simulink model "hcu_main_ADASwEPS"  (Simulink 8.2)
settings: Solver=FixedStepDiscrete  StartTime=0.0  StopTime=inf  FixedStep=0.001  RelTol=1e-3
PostLoadFcn:
  | , if any(exist('dsrtsu_mdlpostloadfcn', 'file') == [2, 3, 6]), try dsrtsu_mdlpostloadfcn('Execute', bdroot); catch fprintf('Error in PostLoadFcn (dsrtsu_mdlpostloadfcn) for model "%s":\n %s\n', bdroot, lasterr); end, end,
values from neighbouring files (symbols this model uses):
  C_TASK_1MS_S = (	C_TICK_TIME_S       )    [hcu_local_hdr.m]    (also in temp_ovrd_values.m = double(	0.001                  ))
  C_TICK_TIME_S = single(	0.005	    	)    [hcu_local_hdr.m]
  ENUM_EPSLFCSTATUS_ACTIVE = uint8(  2  )    [hcu_local_hdr.m]
  ENUM_EPSLFCSTATUS_TRANSITION = uint8(  3  )    [hcu_local_hdr.m]
  ENUM_EPSLKASTATUS_ACTIVE = uint8(  2  )    [hcu_local_hdr.m]
  ENUM_EPSMODEREQ_ANGLE = uint8(  1  )    [hcu_local_hdr.m]
  ENUM_EPSMODEREQ_INTERNAL = uint8(  0  )    [hcu_local_hdr.m]
  ENUM_EPSMODEREQ_TORQUE = uint8(  2  )    [hcu_local_hdr.m]
  ENUM_GEARPOSN_1ST = uint8(  1  )    [hcu_local_hdr.m]
  ENUM_GEARPOSN_2ND = uint8(  2  )    [hcu_local_hdr.m]
  ENUM_GEARPOSN_3RD = uint8(  3  )    [hcu_local_hdr.m]
  ENUM_GEARPOSN_4TH = uint8(  4  )    [hcu_local_hdr.m]
  ENUM_GEARPOSN_5TH = uint8(  5  )    [hcu_local_hdr.m]
  ENUM_GEARPOSN_6TH = uint8(  6  )    [hcu_local_hdr.m]
  ENUM_GEARPOSN_R = uint8(  7  )    [hcu_local_hdr.m]
  FALSE = boolean( 0 )    [hcu_local_hdr.m]
  TRUE = boolean( 1 )    [hcu_local_hdr.m]
undefined symbols (not defined in the file or in its folder): AISP_EPSCurrent_pct, AISP_TqASensorDelta_pct, AISP_TqBSensorDelta_pct, dHAL_IN, hal, INVALID_ABS1_TIMEOUT, INVALID_ABS2_TIMEOUT, INVALID_ABS3_TIMEOUT, INVALID_ABS4_TIMEOUT, INVALID_AC1_TIMEOUT, INVALID_ADASTORQ_REQ, INVALID_BCM1_TIMEOUT, INVALID_BCM2_TIMEOUT, INVALID_BOOSTER_VAC, INVALID_CSW1_TIMEOUT, INVALID_CUR_VEHDECE, INVALID_CURBRAKEDECE_REQ, INVALID_CURSTEERANG_REQ, INVALID_CURSTEERTQ_REQ, INVALID_ECM1_TIMEOUT, INVALID_ECM2_TIMEOUT, INVALID_ECM3_TIMEOUT, INVALID_ECM9_TIMEOUT, INVALID_ENG_TORQUE_FRICTIONAL, INVALID_ENG_TORQUE_INDICATED, INVALID_ENG_TORQUE_INDICATEDCOR, INVALID_ENG_TQ_MAX, INVALID_ENG_TQ_MIN, INVALID_EPAS2_TIMEOUT, INVALID_EPAS3_TIMEOUT, INVALID_EPB1_TIMEOUT, INVALID_EPS_BATTVOLT, INVALID_ESC_BATTVOLT, INVALID_GRADE, INVALID_HCU3_TIMEOUT, INVALID_HCU4_TIMEOUT, INVALID_HMI1_TIMEOUT, INVALID_HMI2_TIMEOUT, INVALID_LAT_ACC, INVALID_LONG_ACC, INVALID_MC_PRESSURE, INVALID_METER1_TIMEOUT, INVALID_METER3_TIMEOUT, INVALID_METER_VEHSPD, INVALID_ODO_METER, INVALID_OUTSIDE_TEMP, INVALID_PARKBRAKEBIND_STAT, INVALID_PEDALTQ_REQ, INVALID_SAS1_TIMEOUT, INVALID_SAS_ANGLE, INVALID_SHIFTER_POSN, INVALID_TCM1_TIMEOUT, INVALID_TCM2_TIMEOUT, INVALID_VCU1_TIMEOUT, INVALID_VCU2_TIMEOUT, INVALID_VEH_CRASH, INVALID_VEH_SPD, INVALID_WHEEL_SPD, INVALID_YAW_RATE, KHAL_MssgIdObj1_num ... (+8)
libraries: simulink x147, hcu_lib x38, rti1401lib_dio_type3 x4, rtimmsu_dsrtlib x3, app x1, rtiethernetudplib x1, rti1401lib_adc_type4 x1, rti1401lib_dac_type3 x1, inp x1, lidr x1, outp x1
(part 10 of 15)

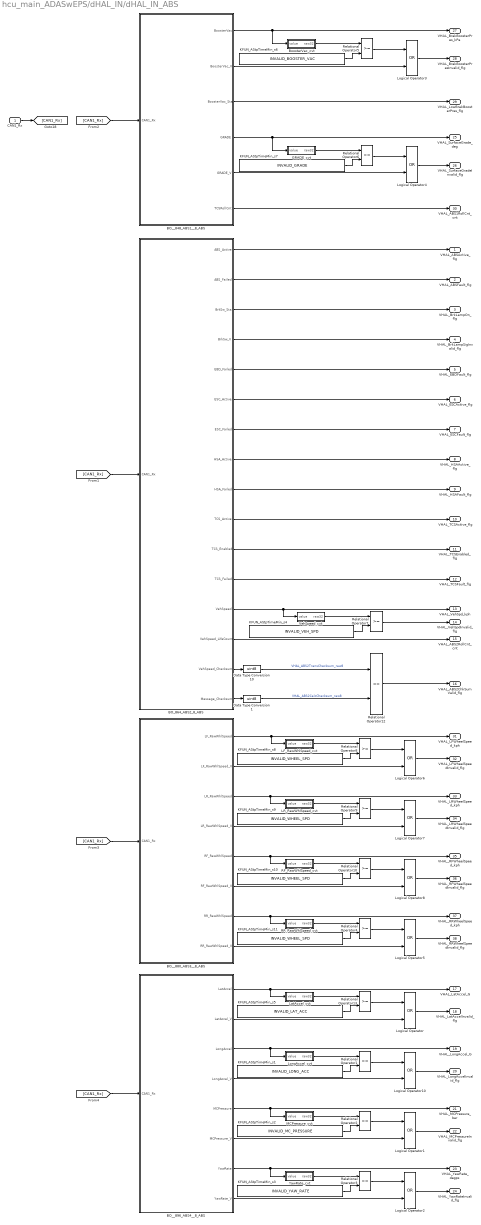
== system hcu_main_ADASwEPS/dHAL_IN/dHAL_IN_ABS ==
  CAN1_Rx : Inport
  BO_864_ABS2_8_ABS : Subsystem
  BO__848_ABS1__8_ABS : Subsystem
  BO__880_ABS3__8_ABS : Subsystem
  BO__896_ABS4__8_ABS : Subsystem
  BoosterVac_cvt : Subsystem  mask(ConvertOut){gain=0.3937, offset=0}
      mask help:
      | Conversion Formula
      |
      | The conversion formula is
      |
      | raw_value = (physical_value - Offset) / Factor
      |
      | where physical_value is the value of the signal after it is saturated using the specified Min and Max values. raw_value is the packed signal value.
  Data Type Conversion1 : DataTypeConversion  OutDataTypeStr=uint8
  Data Type Conversion10 : DataTypeConversion  OutDataTypeStr=uint8
  GRADE_cvt : Subsystem  mask(ConvertOut){gain=0.354331, offset=-45}
      mask help:
      | Conversion Formula
      |
      | The conversion formula is
      |
      | raw_value = (physical_value - Offset) / Factor
      |
      | where physical_value is the value of the signal after it is saturated using the specified Min and Max values. raw_value is the packed signal value.
  KFUN_AStpTimeMin_s1 : Constant  Value=INVALID_LONG_ACC
  KFUN_AStpTimeMin_s{8..11} (4 alike) : Constant  Value=INVALID_WHEEL_SPD
  KFUN_AStpTimeMin_s2 : Constant  Value=INVALID_MC_PRESSURE
  KFUN_AStpTimeMin_s3 : Constant  Value=INVALID_YAW_RATE
  KFUN_AStpTimeMin_s4 : Constant  Value=INVALID_VEH_SPD
  KFUN_AStpTimeMin_s5 : Constant  Value=INVALID_LAT_ACC
  KFUN_AStpTimeMin_s6 : Constant  Value=INVALID_BOOSTER_VAC
  KFUN_AStpTimeMin_s7 : Constant  Value=INVALID_GRADE
  LF_RawWhlSpeed_cvt : Subsystem  mask(ConvertOut){gain=0.015625, offset=0}
      mask help:
      | Conversion Formula
      |
      | The conversion formula is
      |
      | raw_value = (physical_value - Offset) / Factor
      |
      | where physical_value is the value of the signal after it is saturated using the specified Min and Max values. raw_value is the packed signal value.
  LR_RawWhlSpeed_cvt : Subsystem  mask(ConvertOut){gain=0.015625, offset=0}
      mask help:
      | Conversion Formula
      |
      | The conversion formula is
      |
      | raw_value = (physical_value - Offset) / Factor
      |
      | where physical_value is the value of the signal after it is saturated using the specified Min and Max values. raw_value is the packed signal value.
  LatAccel_cvt : Subsystem  mask(ConvertOut){gain=0.01, offset=-1.27}
      mask help:
      | Conversion Formula
      |
      | The conversion formula is
      |
      | raw_value = (physical_value - Offset) / Factor
      |
      | where physical_value is the value of the signal after it is saturated using the specified Min and Max values. raw_value is the packed signal value.
  Logical Operator{,1..8,10} (10 alike) : Logic  Operator=OR  AllPortsSameDT=off  OutDataTypeStr=boolean
  LongAccel_cvt : Subsystem  mask(ConvertOut){gain=0.01, offset=-1.27}
      mask help:
      | Conversion Formula
      |
      | The conversion formula is
      |
      | raw_value = (physical_value - Offset) / Factor
      |
      | where physical_value is the value of the signal after it is saturated using the specified Min and Max values. raw_value is the packed signal value.
  MCPressure_cvt : Subsystem  mask(ConvertOut){gain=0.1, offset=-11.6}
      mask help:
      | Conversion Formula
      |
      | The conversion formula is
      |
      | raw_value = (physical_value - Offset) / Factor
      |
      | where physical_value is the value of the signal after it is saturated using the specified Min and Max values. raw_value is the packed signal value.
  RF_RawWhlSpeed_cvt : Subsystem  mask(ConvertOut){gain=0.015625, offset=0}
      mask help:
      | Conversion Formula
      |
      | The conversion formula is
      |
      | raw_value = (physical_value - Offset) / Factor
      |
      | where physical_value is the value of the signal after it is saturated using the specified Min and Max values. raw_value is the packed signal value.
  RR_RawWhlSpeed_cvt : Subsystem  mask(ConvertOut){gain=0.015625, offset=0}
      mask help:
      | Conversion Formula
      |
      | The conversion formula is
      |
      | raw_value = (physical_value - Offset) / Factor
      |
      | where physical_value is the value of the signal after it is saturated using the specified Min and Max values. raw_value is the packed signal value.
  Relational Operator{1..10,13} (11 alike) : RelationalOperator  OutDataTypeStr=boolean
  Relational Operator12 : RelationalOperator  Operator===  OutDataTypeStr=boolean
  VehSpeed_cvt : Subsystem  mask(ConvertOut){gain=0.125, offset=0}
      mask help:
      | Conversion Formula
      |
      | The conversion formula is
      |
      | raw_value = (physical_value - Offset) / Factor
      |
      | where physical_value is the value of the signal after it is saturated using the specified Min and Max values. raw_value is the packed signal value.
  YawRate_cvt : Subsystem  mask(ConvertOut){gain=0.1, offset=-100}
      mask help:
      | Conversion Formula
      |
      | The conversion formula is
      |
      | raw_value = (physical_value - Offset) / Factor
      |
      | where physical_value is the value of the signal after it is saturated using the specified Min and Max values. raw_value is the packed signal value.
  VHAL_ABSActive_flg : Outport
  VHAL_ABSFault_flg : Outport  Port=2
  VHAL_BrkLampOn_flg : Outport  Port=3
  VHAL_BrkLampSigInvalid_flg : Outport  Port=4
  VHAL_EBDFault_flg : Outport  Port=5
  VHAL_ESCActive_flg : Outport  Port=6
  VHAL_ESCFault_flg : Outport  Port=7
  VHAL_HSAActive_flg : Outport  Port=8
  VHAL_HSAFault_flg : Outport  Port=9
  VHAL_TCSActive_flg : Outport  Port=10
  VHAL_TCSEnabled_flg : Outport  Port=11
  VHAL_TCSFault_flg : Outport  Port=12
  VHAL_VehSpd_kph : Outport  Port=13
  VHAL_VehSpdInvalid_flg : Outport  Port=14
  VHAL_ABS2RollCnt_cnt : Outport  Port=15
  VHAL_ABS2ChkSumValid_flg : Outport  Port=16
  VHAL_LatAccel_G : Outport  Port=17
  VHAL_LatAccelInvalid_flg : Outport  Port=18
  VHAL_LongAccel_G : Outport  Port=19
  VHAL_LongAccelInvalid_flg : Outport  Port=20
  VHAL_MCPressure_bar : Outport  Port=21
  VHAL_MCPressureInvalid_flg : Outport  Port=22
  VHAL_YawRate_degps : Outport  Port=23
  VHAL_YawRateInvalid_flg : Outport  Port=24
  VHAL_SurfaceGrade_deg : Outport  Port=25
  VHAL_SurfaceGradeInvalid_flg : Outport  Port=26
  VHAL_BrakBoosterPres_kPa : Outport  Port=27
  VHAL_BrakBoosterPresInvalid_flg : Outport  Port=28
  VHAL_LowBrakBoosterPres_flg : Outport  Port=29
  VHAL_ABS1RollCnt_cnt : Outport  Port=30
  VHAL_LFWheelSpeed_kph : Outport  Port=31
  VHAL_LFWheelSpeedInvalid_flg : Outport  Port=32
  VHAL_LRWheelSpeed_kph : Outport  Port=33
  VHAL_LRWheelSpeedInvalid_flg : Outport  Port=34
  VHAL_RFWheelSpeed_kph : Outport  Port=35
  VHAL_RFWheelSpeedInvalid_flg : Outport  Port=36
  VHAL_RRWheelSpeed_kph : Outport  Port=37
  VHAL_RRWheelSpeedInvalid_flg : Outport  Port=38
  wires:
  BO_864_ABS2_8_ABS/1(ABS_Active) -> VHAL_ABSActive_flg/1
  BO_864_ABS2_8_ABS/2(ABS_Failed) -> VHAL_ABSFault_flg/1
  BO_864_ABS2_8_ABS/3(BrkSw_Sta) -> VHAL_BrkLampOn_flg/1
  BO_864_ABS2_8_ABS/4(BrkSw_V) -> VHAL_BrkLampSigInvalid_flg/1
  BO_864_ABS2_8_ABS/5(EBD_Failed) -> VHAL_EBDFault_flg/1
  BO_864_ABS2_8_ABS/6(ESC_Active) -> VHAL_ESCActive_flg/1
  BO_864_ABS2_8_ABS/7(ESC_Failed) -> VHAL_ESCFault_flg/1
  BO_864_ABS2_8_ABS/10(TCS_Active) -> VHAL_TCSActive_flg/1
  BO_864_ABS2_8_ABS/11(TCS_Enabled) -> VHAL_TCSEnabled_flg/1
  BO_864_ABS2_8_ABS/12(TCS_Failed) -> VHAL_TCSFault_flg/1
  BO__848_ABS1__8_ABS/6(TCSRollCnt) -> VHAL_ABS1RollCnt_cnt/1
  BO__896_ABS4__8_ABS/2(LatAccel_V) -> Logical Operator/2
  BO__896_ABS4__8_ABS/6(MCPressure_V) -> Logical Operator1/2
  Logical Operator/1 -> VHAL_LatAccelInvalid_flg/1
  Logical Operator10/1 -> VHAL_LongAccelInvalid_flg/1
  Logical Operator1/1 -> VHAL_MCPressureInvalid_flg/1
  Logical Operator2/1 -> VHAL_YawRateInvalid_flg/1
  BO_864_ABS2_8_ABS/8(HSA_Active) -> VHAL_HSAActive_flg/1
  BO_864_ABS2_8_ABS/9(HSA_Failed) -> VHAL_HSAFault_flg/1
  BO__848_ABS1__8_ABS/3(BoosterVac_Sta) -> VHAL_LowBrakBoosterPres_flg/1
  BO__880_ABS3__8_ABS/8(RR_RawWhlSpeed_V) -> Logical Operator5/2
  Logical Operator5/1 -> VHAL_RRWheelSpeedInvalid_flg/1
  BO_864_ABS2_8_ABS/14(VehSpeed_LifeCount) -> VHAL_ABS2RollCnt_cnt/1
  BO_864_ABS2_8_ABS/15(VehSpeed_Checksum) -> Data Type Conversion10/1
  BO_864_ABS2_8_ABS/16(Message_Checksum) -> Data Type Conversion1/1
  Relational Operator12/1 -> VHAL_ABS2ChkSumValid_flg/1
  Data Type Conversion10/1 -> Relational Operator12/1  "VHAL_ABS2TransChecksum_raw8"
  Data Type Conversion1/1 -> Relational Operator12/2  "VHAL_ABS2CalcChecksum_raw8"
  CAN1_Rx/1 -> [CAN1_Rx]
  [CAN1_Rx] -> BO_864_ABS2_8_ABS/1(CAN1_Rx)
  [CAN1_Rx] -> BO__848_ABS1__8_ABS/1(CAN1_Rx)
  [CAN1_Rx] -> BO__880_ABS3__8_ABS/1(CAN1_Rx)
  [CAN1_Rx] -> BO__896_ABS4__8_ABS/1(CAN1_Rx)
  BO__896_ABS4__8_ABS/8(YawRate_V) -> Logical Operator2/2
  BO__896_ABS4__8_ABS/4(LongAccel_V) -> Logical Operator10/2
  BO__896_ABS4__8_ABS/1(LatAccel) -> LatAccel_cvt/1(value), VHAL_LatAccel_G/1
  KFUN_AStpTimeMin_s5/1 -> Relational Operator13/2
  LatAccel_cvt/1(raw32) -> Relational Operator13/1
  Relational Operator13/1 -> Logical Operator/1
  BO__896_ABS4__8_ABS/3(LongAccel) -> LongAccel_cvt/1(value), VHAL_LongAccel_G/1
  KFUN_AStpTimeMin_s1/1 -> Relational Operator1/2
  LongAccel_cvt/1(raw32) -> Relational Operator1/1
  Relational Operator1/1 -> Logical Operator10/1
  BO__896_ABS4__8_ABS/5(MCPressure) -> MCPressure_cvt/1(value), VHAL_MCPressure_bar/1
  KFUN_AStpTimeMin_s2/1 -> Relational Operator2/2
  MCPressure_cvt/1(raw32) -> Relational Operator2/1
  Relational Operator2/1 -> Logical Operator1/1
  BO__896_ABS4__8_ABS/7(YawRate) -> YawRate_cvt/1(value), VHAL_YawRate_degps/1
  KFUN_AStpTimeMin_s3/1 -> Relational Operator3/2
  YawRate_cvt/1(raw32) -> Relational Operator3/1
  Relational Operator3/1 -> Logical Operator2/1
  BO__848_ABS1__8_ABS/2(BoosterVac_V) -> Logical Operator3/2
  Logical Operator3/1 -> VHAL_BrakBoosterPresInvalid_flg/1
  BO__848_ABS1__8_ABS/1(BoosterVac) -> BoosterVac_cvt/1(value), VHAL_BrakBoosterPres_kPa/1
  KFUN_AStpTimeMin_s6/1 -> Relational Operator5/2
  BoosterVac_cvt/1(raw32) -> Relational Operator5/1
  Relational Operator5/1 -> Logical Operator3/1
  Logical Operator4/1 -> VHAL_SurfaceGradeInvalid_flg/1
  BO__848_ABS1__8_ABS/4(GRADE) -> GRADE_cvt/1(value), VHAL_SurfaceGrade_deg/1
  KFUN_AStpTimeMin_s7/1 -> Relational Operator6/2
  GRADE_cvt/1(raw32) -> Relational Operator6/1
  Relational Operator6/1 -> Logical Operator4/1
  BO__848_ABS1__8_ABS/5(GRADE_V) -> Logical Operator4/2
  BO_864_ABS2_8_ABS/13(VehSpeed) -> VehSpeed_cvt/1(value), VHAL_VehSpd_kph/1
  KFUN_AStpTimeMin_s4/1 -> Relational Operator7/2
  VehSpeed_cvt/1(raw32) -> Relational Operator7/1
  Relational Operator7/1 -> VHAL_VehSpdInvalid_flg/1
  BO__880_ABS3__8_ABS/7(RR_RawWhlSpeed) -> RR_RawWhlSpeed_cvt/1(value), VHAL_RRWheelSpeed_kph/1
  KFUN_AStpTimeMin_s11/1 -> Relational Operator4/2
  RR_RawWhlSpeed_cvt/1(raw32) -> Relational Operator4/1
  Relational Operator4/1 -> Logical Operator5/1
  BO__880_ABS3__8_ABS/5(RF_RawWhlSpeed) -> RF_RawWhlSpeed_cvt/1(value), VHAL_RFWheelSpeed_kph/1
  KFUN_AStpTimeMin_s10/1 -> Relational Operator10/2
  RF_RawWhlSpeed_cvt/1(raw32) -> Relational Operator10/1
  Relational Operator10/1 -> Logical Operator8/1
  BO__880_ABS3__8_ABS/6(RF_RawWhlSpeed_V) -> Logical Operator8/2
  Logical Operator8/1 -> VHAL_RFWheelSpeedInvalid_flg/1
  BO__880_ABS3__8_ABS/3(LR_RawWhlSpeed) -> LR_RawWhlSpeed_cvt/1(value), VHAL_LRWheelSpeed_kph/1
  KFUN_AStpTimeMin_s9/1 -> Relational Operator9/2
  LR_RawWhlSpeed_cvt/1(raw32) -> Relational Operator9/1
  Relational Operator9/1 -> Logical Operator7/1
  BO__880_ABS3__8_ABS/4(LR_RawWhlSpeed_V) -> Logical Operator7/2
  Logical Operator7/1 -> VHAL_LRWheelSpeedInvalid_flg/1
  BO__880_ABS3__8_ABS/1(LF_RawWhlSpeed) -> LF_RawWhlSpeed_cvt/1(value), VHAL_LFWheelSpeed_kph/1
  KFUN_AStpTimeMin_s8/1 -> Relational Operator8/2
  LF_RawWhlSpeed_cvt/1(raw32) -> Relational Operator8/1
  Relational Operator8/1 -> Logical Operator6/1
  Logical Operator6/1 -> VHAL_LFWheelSpeedInvalid_flg/1
  BO__880_ABS3__8_ABS/2(LF_RawWhlSpeed_V) -> Logical Operator6/2

== system hcu_main_ADASwEPS/dHAL_IN/dHAL_IN_AC ==
  CAN1_Rx : Inport
  BO__1120_AC1__8_AC : Subsystem
  KFUN_AStpTimeMin_s1 : Constant  Value=INVALID_OUTSIDE_TEMP
  Relational Operator4 : RelationalOperator  OutDataTypeStr=boolean
  Sta_Out_Temp_cvt : Subsystem  mask(ConvertOut){gain=1, offset=-40}
      mask help:
      | Conversion Formula
      |
      | The conversion formula is
      |
      | raw_value = (physical_value - Offset) / Factor
      |
      | where physical_value is the value of the signal after it is saturated using the specified Min and Max values. raw_value is the packed signal value.
  VHAL_OutsideTemp_degC : Outport
  VHAL_OutsideTempInvalid_flg : Outport  Port=2
  wires:
  CAN1_Rx/1 -> [CAN1_Rx]
  [CAN1_Rx] -> BO__1120_AC1__8_AC/1(CAN1_Rx)
  BO__1120_AC1__8_AC/1(Sta_Out_Temp) -> Sta_Out_Temp_cvt/1(value), VHAL_OutsideTemp_degC/1
  KFUN_AStpTimeMin_s1/1 -> Relational Operator4/2
  Sta_Out_Temp_cvt/1(raw32) -> Relational Operator4/1
  Relational Operator4/1 -> VHAL_OutsideTempInvalid_flg/1

== system hcu_main_ADASwEPS/dHAL_IN/dHAL_IN_BCM ==
  CAN1_Rx : Inport
  BO__1008_BCM2__8_BCM : Subsystem
  BO__1056_BCM1__8_BCM : Subsystem
  Compare To Constant : simulink/Logic and Bit Operations/Compare To Constant  relop===  const=5  OutDataTypeStr=boolean  ZeroCross=off
  Compare To Constant1 : simulink/Logic and Bit Operations/Compare To Constant  relop=~=  const=5  OutDataTypeStr=boolean  ZeroCross=off
  Compare To Constant2 : simulink/Logic and Bit Operations/Compare To Constant  relop=~=  const=0  OutDataTypeStr=boolean  ZeroCross=off
  KFUN_AStpTimeMin_s3 : Constant  Value=INVALID_VEH_CRASH
  Logical Operator : Logic  Operator=OR  AllPortsSameDT=off  OutDataTypeStr=boolean
  Logical Operator1 : Logic  AllPortsSameDT=off  OutDataTypeStr=boolean
  Relational Operator3 : RelationalOperator  Operator===  OutDataTypeStr=boolean
  VHAL_KeySwitchStatus_enum : Outport
  VHAL_TurnSignalSwL_flg : Outport  Port=2
  VHAL_TurnSignalSwR_flg : Outport  Port=3
  VHAL_DriverDoorOpen_flg : Outport  Port=4
  VHAL_PassengerDoorOpen_flg : Outport  Port=5
  VHAL_LRDoorOpen_flg : Outport  Port=6
  VHAL_RRDoorOpen_flg : Outport  Port=7
  VHAL_TailGateOpen_flg : Outport  Port=8
  VHAL_AnyDoorOpen_flg : Outport  Port=9
  VHAL_HazardLightSw_flg : Outport  Port=10
  VHAL_VehCrashed_flg : Outport  Port=11
  VHAL_VehCrashedInvalid_flg : Outport  Port=12
  wires:
  Logical Operator/1 -> VHAL_VehCrashedInvalid_flg/1
  Relational Operator3/1 -> Logical Operator/1
  KFUN_AStpTimeMin_s3/1 -> Relational Operator3/2
  Compare To Constant/1 -> VHAL_VehCrashed_flg/1
  BO__1008_BCM2__8_BCM/1(BCM_SRS_Crash_Info) -> Compare To Constant2/1, Compare To Constant1/1, Relational Operator3/1, Compare To Constant/1
  BO__1056_BCM1__8_BCM/3(BCM_Hazard_Sta) -> VHAL_HazardLightSw_flg/1
  BO__1056_BCM1__8_BCM/1(BCM_AllDrSw_Sta) -> VHAL_AnyDoorOpen_flg/1
  BO__1056_BCM1__8_BCM/10(BCM_TGateSw_Sta) -> VHAL_TailGateOpen_flg/1
  BO__1056_BCM1__8_BCM/8(BCM_RRDrSw_Sta) -> VHAL_RRDoorOpen_flg/1
  BO__1056_BCM1__8_BCM/5(BCM_LRDrSw_Sta) -> VHAL_LRDoorOpen_flg/1
  BO__1056_BCM1__8_BCM/7(BCM_PDrSw_Sta) -> VHAL_PassengerDoorOpen_flg/1
  BO__1056_BCM1__8_BCM/2(BCM_DDrSw_Sta) -> VHAL_DriverDoorOpen_flg/1
  BO__1056_BCM1__8_BCM/4(BCM_Key_Sta) -> VHAL_KeySwitchStatus_enum/1
  BO__1056_BCM1__8_BCM/9(BCM_RTurnLp_Sta) -> VHAL_TurnSignalSwR_flg/1
  BO__1056_BCM1__8_BCM/6(BCM_LTurnLp_Sta) -> VHAL_TurnSignalSwL_flg/1
  CAN1_Rx/1 -> [CAN1_Rx]
  [CAN1_Rx] -> BO__1056_BCM1__8_BCM/1(CAN1_Rx)
  [CAN1_Rx] -> BO__1008_BCM2__8_BCM/1(CAN1_Rx)
  Compare To Constant1/1 -> Logical Operator1/1
  Compare To Constant2/1 -> Logical Operator1/2
  Logical Operator1/1 -> Logical Operator/2

== system hcu_main_ADASwEPS/dHAL_IN/dHAL_IN_ECM ==
  CAN1_Rx : Inport
  BO_790_ECM1_8_ECM : Subsystem
  BO_809_ECM2_8_ECM : Subsystem
  BO_821_ECM3_8_ECM : Subsystem
  BO_875_ECM9_8_ECM : Subsystem
  CAN_TQFR_cvt : Subsystem  mask(ConvertOut){gain=1.96, offset=-100}
      mask help:
      | Conversion Formula
      |
      | The conversion formula is
      |
      | raw_value = (physical_value - Offset) / Factor
      |
      | where physical_value is the value of the signal after it is saturated using the specified Min and Max values. raw_value is the packed signal value.
  CAN_TQI_ACOR_cvt : Subsystem  mask(ConvertOut){gain=1.96, offset=-100}
      mask help:
      | Conversion Formula
      |
      | The conversion formula is
      |
      | raw_value = (physical_value - Offset) / Factor
      |
      | where physical_value is the value of the signal after it is saturated using the specified Min and Max values. raw_value is the packed signal value.
  CAN_TQI_cvt : Subsystem  mask(ConvertOut){gain=1.96, offset=-100}
      mask help:
      | Conversion Formula
      |
      | The conversion formula is
      |
      | raw_value = (physical_value - Offset) / Factor
      |
      | where physical_value is the value of the signal after it is saturated using the specified Min and Max values. raw_value is the packed signal value.
  EngTqMax_cvt : Subsystem  mask(ConvertOut){gain=0.0078, offset=-100}
      mask help:
      | Conversion Formula
      |
      | The conversion formula is
      |
      | raw_value = (physical_value - Offset) / Factor
      |
      | where physical_value is the value of the signal after it is saturated using the specified Min and Max values. raw_value is the packed signal value.
  EngTqMin_cvt : Subsystem  mask(ConvertOut){gain=0.0078, offset=-100}
      mask help:
      | Conversion Formula
      |
      | The conversion formula is
      |
      | raw_value = (physical_value - Offset) / Factor
      |
      | where physical_value is the value of the signal after it is saturated using the specified Min and Max values. raw_value is the packed signal value.
  KFUN_AStpTimeMin_s1 : Constant  Value=INVALID_ENG_TORQUE_INDICATED
  KFUN_AStpTimeMin_s2 : Constant  Value=INVALID_ENG_TORQUE_INDICATEDCOR
  KFUN_AStpTimeMin_s3 : Constant  Value=INVALID_ENG_TORQUE_FRICTIONAL
  KFUN_AStpTimeMin_s5 : Constant  Value=INVALID_ENG_TQ_MAX
  KFUN_AStpTimeMin_s6 : Constant  Value=INVALID_ENG_TQ_MIN
  Relational Operator{1..5} (5 alike) : RelationalOperator  OutDataTypeStr=boolean
  VHAL_AccelPedalPosn_pct : Outport
  VHAL_AccelPedalPosnInvalid_flg : Outport  Port=2
  VHAL_EffAccelPedalPosn_pct : Outport  Port=3
  VHAL_EffAccelPedalPosnInvalid_flg : Outport  Port=4
  VHAL_EngSpd_rpm : Outport  Port=5
  VHAL_EngSpdInvalid_flg : Outport  Port=6
  VHAL_EngTqIndicated_Nm : Outport  Port=7
  VHAL_EngTqIndicatedInvalid_flg : Outport  Port=8
  VHAL_EngTqIndicatedCOR_Nm : Outport  Port=9
  VHAL_EngTqIndicatedCORInvalid_flg : Outport  Port=10
  VHAL_EngTqUnCORFault_flg : Outport  Port=11
  VHAL_EngTqFriction_Nm : Outport  Port=12
  VHAL_EngTqFrictionInvalid_flg : Outport  Port=13
  VHAL_EngTqMax_Nm : Outport  Port=14
  VHAL_EngTqMaxInvalid_flg : Outport  Port=15
  VHAL_EngTqMin_Nm : Outport  Port=16
  VHAL_EngTqMinInvalid_flg : Outport  Port=17
  VHAL_EMSHybridOpState_enum : Outport  Port=18
  VHAL_EMSOpState_enum : Outport  Port=19
  VHAL_ECM9RollCnt_cnt : Outport  Port=20
  VHAL_EngHoodOpen_flg : Outport  Port=21
  VHAL_OBDWarnCycAchiv_flg : Outport  Port=22
  VHAL_OBDDriveCycAchiv_flg : Outport  Port=23
  wires:
  CAN1_Rx/1 -> [CAN1_Rx]
  [CAN1_Rx] -> BO_821_ECM3_8_ECM/1(CAN1_Rx)
  BO_821_ECM3_8_ECM/4(LV_CAN_ERRPVS) -> VHAL_EffAccelPedalPosnInvalid_flg/1
  BO_821_ECM3_8_ECM/3(LV_CAN_ERRPAS) -> VHAL_AccelPedalPosnInvalid_flg/1
  BO_821_ECM3_8_ECM/2(CAN_PV_EFC) -> VHAL_EffAccelPedalPosn_pct/1
  BO_821_ECM3_8_ECM/1(CAN_PV_AV) -> VHAL_AccelPedalPosn_pct/1
  [CAN1_Rx] -> BO_790_ECM1_8_ECM/1(CAN1_Rx)
  BO_790_ECM1_8_ECM/6(LV_CAN_SUB_TQI) -> VHAL_EngTqUnCORFault_flg/1
  Relational Operator2/1 -> VHAL_EngTqIndicatedCORInvalid_flg/1
  BO_790_ECM1_8_ECM/4(CAN_TQI_ACOR) -> VHAL_EngTqIndicatedCOR_Nm/1, CAN_TQI_ACOR_cvt/1(value)
  BO_790_ECM1_8_ECM/3(CAN_TQI) -> VHAL_EngTqIndicated_Nm/1, CAN_TQI_cvt/1(value)
  Relational Operator1/1 -> VHAL_EngTqIndicatedInvalid_flg/1
  BO_790_ECM1_8_ECM/1(CAN_N) -> VHAL_EngSpd_rpm/1
  BO_790_ECM1_8_ECM/5(LV_CAN_N_ERR) -> VHAL_EngSpdInvalid_flg/1
  BO_790_ECM1_8_ECM/2(CAN_TQFR) -> VHAL_EngTqFriction_Nm/1, CAN_TQFR_cvt/1(value)
  Relational Operator3/1 -> VHAL_EngTqFrictionInvalid_flg/1
  [CAN1_Rx] -> BO_875_ECM9_8_ECM/1(CAN1_Rx1)
  BO_875_ECM9_8_ECM/3(EMSOpState) -> VHAL_EMSOpState_enum/1
  BO_875_ECM9_8_ECM/2(EMSHybridOpState) -> VHAL_EMSHybridOpState_enum/1
  BO_875_ECM9_8_ECM/1(ECM9RollCnt) -> VHAL_ECM9RollCnt_cnt/1
  [CAN1_Rx] -> BO_809_ECM2_8_ECM/1(CAN1_Rx)
  BO_809_ECM2_8_ECM/2(CAN_OBD_STAT_WU) -> VHAL_OBDWarnCycAchiv_flg/1
  BO_809_ECM2_8_ECM/1(Eng_Hood_SW) -> VHAL_EngHoodOpen_flg/1
  KFUN_AStpTimeMin_s2/1 -> Relational Operator2/2
  KFUN_AStpTimeMin_s1/1 -> Relational Operator1/2
  KFUN_AStpTimeMin_s3/1 -> Relational Operator3/2
  CAN_TQFR_cvt/1(raw32) -> Relational Operator3/1
  CAN_TQI_cvt/1(raw32) -> Relational Operator1/1
  CAN_TQI_ACOR_cvt/1(raw32) -> Relational Operator2/1
  Relational Operator4/1 -> VHAL_EngTqMaxInvalid_flg/1
  BO_875_ECM9_8_ECM/4(EngTqMax) -> EngTqMax_cvt/1(value), VHAL_EngTqMax_Nm/1
  KFUN_AStpTimeMin_s5/1 -> Relational Operator4/2
  EngTqMax_cvt/1(raw32) -> Relational Operator4/1
  Relational Operator5/1 -> VHAL_EngTqMinInvalid_flg/1
  BO_875_ECM9_8_ECM/5(EngTqMin) -> EngTqMin_cvt/1(value), VHAL_EngTqMin_Nm/1
  KFUN_AStpTimeMin_s6/1 -> Relational Operator5/2
  EngTqMin_cvt/1(raw32) -> Relational Operator5/1
  BO_809_ECM2_8_ECM/3(CAN_OBD_STAT_DR) -> VHAL_OBDDriveCycAchiv_flg/1

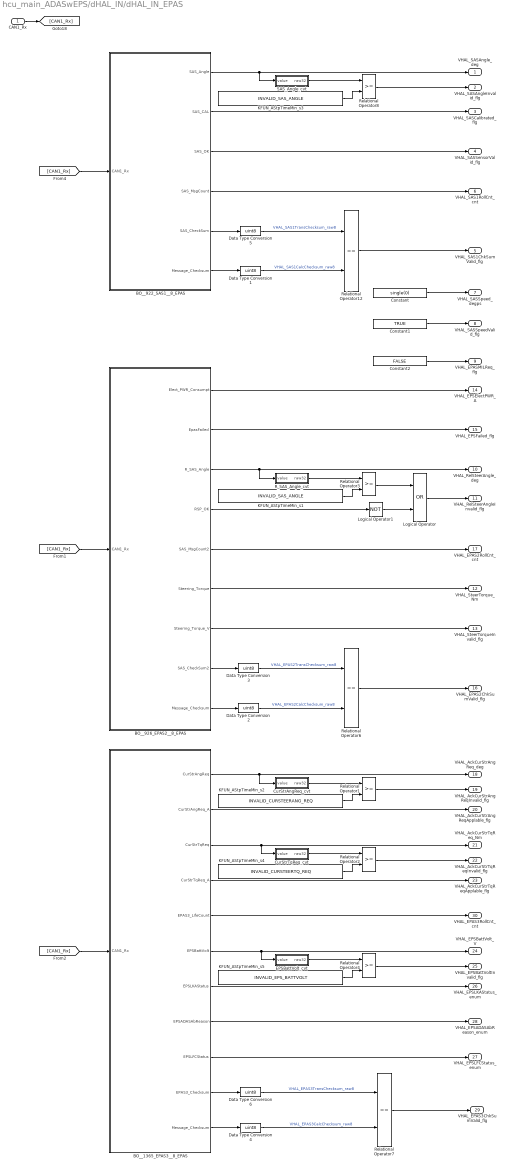
== system hcu_main_ADASwEPS/dHAL_IN/dHAL_IN_EPAS ==
  CAN1_Rx : Inport
  BO__1365_EPAS3__8_EPAS : Subsystem
  BO__922_SAS1__8_EPAS : Subsystem
  BO__926_EPAS2__8_EPAS : Subsystem
  Constant : Constant  Value=single(0)
  Constant1 : Constant  Value=TRUE
  Constant2 : Constant  Value=FALSE
  CurStrAngReq_cvt : Subsystem  mask(ConvertOut){gain=0.1, offset=-720}
      mask help:
      | Conversion Formula
      |
      | The conversion formula is
      |
      | raw_value = (physical_value - Offset) / Factor
      |
      | where physical_value is the value of the signal after it is saturated using the specified Min and Max values. raw_value is the packed signal value.
  CurStrTqReq_cvt : Subsystem  mask(ConvertOut){gain=0.1, offset=-10}
      mask help:
      | Conversion Formula
      |
      | The conversion formula is
      |
      | raw_value = (physical_value - Offset) / Factor
      |
      | where physical_value is the value of the signal after it is saturated using the specified Min and Max values. raw_value is the packed signal value.
  Data Type Conversion{1..6} (6 alike) : DataTypeConversion  OutDataTypeStr=uint8
  EPSBattVolt_cvt : Subsystem  mask(ConvertOut){gain=0.1, offset=0}
      mask help:
      | Conversion Formula
      |
      | The conversion formula is
      |
      | raw_value = (physical_value - Offset) / Factor
      |
      | where physical_value is the value of the signal after it is saturated using the specified Min and Max values. raw_value is the packed signal value.
  KFUN_AStpTimeMin_s1 : Constant  Value=INVALID_SAS_ANGLE
  KFUN_AStpTimeMin_s2 : Constant  Value=INVALID_CURSTEERANG_REQ
  KFUN_AStpTimeMin_s3 : Constant  Value=INVALID_SAS_ANGLE
  KFUN_AStpTimeMin_s4 : Constant  Value=INVALID_CURSTEERTQ_REQ
  KFUN_AStpTimeMin_s5 : Constant  Value=INVALID_EPS_BATTVOLT
  Logical Operator : Logic  Operator=OR  AllPortsSameDT=off  OutDataTypeStr=boolean
  Logical Operator1 : Logic  Operator=NOT  AllPortsSameDT=off  OutDataTypeStr=boolean
  R_SAS_Angle_cvt : Subsystem  mask(ConvertOut){gain=0.1, offset=-1400}
      mask help:
      | Conversion Formula
      |
      | The conversion formula is
      |
      | raw_value = (physical_value - Offset) / Factor
      |
      | where physical_value is the value of the signal after it is saturated using the specified Min and Max values. raw_value is the packed signal value.
  Relational Operator{1..4,8} (5 alike) : RelationalOperator  OutDataTypeStr=boolean
  Relational Operator12 : RelationalOperator  Operator===  OutDataTypeStr=boolean
  Relational Operator6 : RelationalOperator  Operator===  OutDataTypeStr=boolean
  Relational Operator7 : RelationalOperator  Operator===  OutDataTypeStr=boolean
  SAS_Angle_cvt : Subsystem  mask(ConvertOut){gain=0.1, offset=-900}
      mask help:
      | Conversion Formula
      |
      | The conversion formula is
      |
      | raw_value = (physical_value - Offset) / Factor
      |
      | where physical_value is the value of the signal after it is saturated using the specified Min and Max values. raw_value is the packed signal value.
  VHAL_SASAngle_deg : Outport
  VHAL_SASAngleInvalid_flg : Outport  Port=2
  VHAL_SASCalibrated_flg : Outport  Port=3
  VHAL_SASSensorValid_flg : Outport  Port=4
  VHAL_SAS1ChkSumValid_flg : Outport  Port=5
  VHAL_SAS1RollCnt_cnt : Outport  Port=6
  VHAL_SASSpeed_degps : Outport  Port=7
  VHAL_SASSpeedValid_flg : Outport  Port=8
  VHAL_EPASMILReq_flg : Outport  Port=9
  VHAL_RelSteerAngle_deg : Outport  Port=10
  VHAL_RelSteerAngleInvalid_flg : Outport  Port=11
  VHAL_SteerTorque_Nm : Outport  Port=12
  VHAL_SteerTorqueInvalid_flg : Outport  Port=13
  VHAL_EPSElectPWR_A : Outport  Port=14
  VHAL_EPSFailed_flg : Outport  Port=15
  VHAL_EPAS2ChkSumValid_flg : Outport  Port=16
  VHAL_EPAS2RollCnt_cnt : Outport  Port=17
  VHAL_AckCurStrAngReq_deg : Outport  Port=18
  VHAL_AckCurStrAngReqInvalid_flg : Outport  Port=19
  VHAL_AckCurStrAngReqApplable_flg : Outport  Port=20
  VHAL_AckCurStrTqReq_Nm : Outport  Port=21
  VHAL_AckCurStrTqReqInvalid_flg : Outport  Port=22
  VHAL_AckCurStrTqReqApplable_flg : Outport  Port=23
  VHAL_EPSBattVolt_V : Outport  Port=24
  VHAL_EPSBattVoltInvalid_flg : Outport  Port=25
  VHAL_EPSLKAStatus_enum : Outport  Port=26
  VHAL_EPSLFCStatus_enum : Outport  Port=27
  VHAL_EPSADASAbReason_enum : Outport  Port=28
  VHAL_EPAS3ChkSumValid_flg : Outport  Port=29
  VHAL_EPAS3RollCnt_cnt : Outport  Port=30
  wires:
  Constant2/1 -> VHAL_EPASMILReq_flg/1
  Constant1/1 -> VHAL_SASSpeedValid_flg/1
  Constant/1 -> VHAL_SASSpeed_degps/1
  BO__922_SAS1__8_EPAS/2(SAS_CAL) -> VHAL_SASCalibrated_flg/1
  BO__922_SAS1__8_EPAS/4(SAS_MsgCount) -> VHAL_SAS1RollCnt_cnt/1
  BO__922_SAS1__8_EPAS/3(SAS_OK) -> VHAL_SASSensorValid_flg/1
  BO__1365_EPAS3__8_EPAS/5(EPAS3_LifeCount) -> VHAL_EPAS3RollCnt_cnt/1
  BO__926_EPAS2__8_EPAS/1(Elect_PWR_Consumpt) -> VHAL_EPSElectPWR_A/1
  BO__926_EPAS2__8_EPAS/2(EpasFailed) -> VHAL_EPSFailed_flg/1
  BO__926_EPAS2__8_EPAS/4(RSP_OK) -> Logical Operator1/1
  BO__926_EPAS2__8_EPAS/5(SAS_MsgCount2) -> VHAL_EPAS2RollCnt_cnt/1
  BO__926_EPAS2__8_EPAS/6(Steering_Torque) -> VHAL_SteerTorque_Nm/1
  BO__926_EPAS2__8_EPAS/7(Steering_Torque_V) -> VHAL_SteerTorqueInvalid_flg/1
  Logical Operator/1 -> VHAL_RelSteerAngleInvalid_flg/1
  Logical Operator1/1 -> Logical Operator/2
  BO__1365_EPAS3__8_EPAS/4(CurStrTqReq_A) -> VHAL_AckCurStrTqReqApplable_flg/1
  BO__922_SAS1__8_EPAS/5(SAS_CheckSum) -> Data Type Conversion5/1
  BO__922_SAS1__8_EPAS/6(Message_Checksum) -> Data Type Conversion1/1
  Data Type Conversion5/1 -> Relational Operator12/1  "VHAL_SAS1TransChecksum_raw8"
  Data Type Conversion1/1 -> Relational Operator12/2  "VHAL_SAS1CalcChecksum_raw8"
  Relational Operator12/1 -> VHAL_SAS1ChkSumValid_flg/1
  Data Type Conversion3/1 -> Relational Operator6/1  "VHAL_EPAS2TransChecksum_raw8"
  Data Type Conversion2/1 -> Relational Operator6/2  "VHAL_EPAS2CalcChecksum_raw8"
  Relational Operator6/1 -> VHAL_EPAS2ChkSumValid_flg/1
  BO__926_EPAS2__8_EPAS/8(SAS_CheckSum2) -> Data Type Conversion3/1
  BO__926_EPAS2__8_EPAS/9(Message_Checksum) -> Data Type Conversion2/1
  Data Type Conversion6/1 -> Relational Operator7/1  "VHAL_EPAS3TransChecksum_raw8"
  Data Type Conversion4/1 -> Relational Operator7/2  "VHAL_EPAS3CalcChecksum_raw8"
  Relational Operator7/1 -> VHAL_EPAS3ChkSumValid_flg/1
  BO__1365_EPAS3__8_EPAS/10(EPAS3_Checksum) -> Data Type Conversion6/1
  BO__1365_EPAS3__8_EPAS/11(Message_Checksum) -> Data Type Conversion4/1
  BO__1365_EPAS3__8_EPAS/2(CurStrAngReq_A) -> VHAL_AckCurStrAngReqApplable_flg/1
  CAN1_Rx/1 -> [CAN1_Rx]
  [CAN1_Rx] -> BO__922_SAS1__8_EPAS/1(CAN1_Rx)
  [CAN1_Rx] -> BO__926_EPAS2__8_EPAS/1(CAN1_Rx)
  [CAN1_Rx] -> BO__1365_EPAS3__8_EPAS/1(CAN1_Rx)
  BO__922_SAS1__8_EPAS/1(SAS_Angle) -> SAS_Angle_cvt/1(value), VHAL_SASAngle_deg/1
  KFUN_AStpTimeMin_s3/1 -> Relational Operator8/2
  SAS_Angle_cvt/1(raw32) -> Relational Operator8/1
  Relational Operator8/1 -> VHAL_SASAngleInvalid_flg/1
  BO__926_EPAS2__8_EPAS/3(R_SAS_Angle) -> R_SAS_Angle_cvt/1(value), VHAL_RelSteerAngle_deg/1
  KFUN_AStpTimeMin_s1/1 -> Relational Operator3/2
  R_SAS_Angle_cvt/1(raw32) -> Relational Operator3/1
  Relational Operator3/1 -> Logical Operator/1
  BO__1365_EPAS3__8_EPAS/1(CurStrAngReq) -> CurStrAngReq_cvt/1(value), VHAL_AckCurStrAngReq_deg/1
  KFUN_AStpTimeMin_s2/1 -> Relational Operator1/2
  CurStrAngReq_cvt/1(raw32) -> Relational Operator1/1
  Relational Operator1/1 -> VHAL_AckCurStrAngReqInvalid_flg/1
  BO__1365_EPAS3__8_EPAS/3(CurStrTqReq) -> CurStrTqReq_cvt/1(value), VHAL_AckCurStrTqReq_Nm/1
  KFUN_AStpTimeMin_s4/1 -> Relational Operator2/2
  CurStrTqReq_cvt/1(raw32) -> Relational Operator2/1
  Relational Operator2/1 -> VHAL_AckCurStrTqReqInvalid_flg/1
  BO__1365_EPAS3__8_EPAS/6(EPSBattVolt) -> EPSBattVolt_cvt/1(value), VHAL_EPSBattVolt_V/1
  KFUN_AStpTimeMin_s5/1 -> Relational Operator4/2
  EPSBattVolt_cvt/1(raw32) -> Relational Operator4/1
  Relational Operator4/1 -> VHAL_EPSBattVoltInvalid_flg/1
  BO__1365_EPAS3__8_EPAS/7(EPSLKAStatus) -> VHAL_EPSLKAStatus_enum/1
  BO__1365_EPAS3__8_EPAS/8(EPSADASAbReason) -> VHAL_EPSADASAbReason_enum/1
  BO__1365_EPAS3__8_EPAS/9(EPSLFCStatus) -> VHAL_EPSLFCStatus_enum/1

== system hcu_main_ADASwEPS/dHAL_IN/dHAL_IN_HWIO ==
  IgnitionVolt_V : Constant  Value=12
  VbatprotVolt_V : Constant  Value=12
  VHAL_IgnitionVolt_V : Outport
  VHAL_VbatprotVolt_V : Outport  Port=2
  wires:
  IgnitionVolt_V/1 -> VHAL_IgnitionVolt_V/1
  VbatprotVolt_V/1 -> VHAL_VbatprotVolt_V/1

== system hcu_main_ADASwEPS/dHAL_IN/dHAL_IN_LLSW ==
  ADCFault_enum : Constant  Value=0
  AppTime_ms : Constant
  BuzzerSwOnFltOpenCircuit_enum : Constant  Value=0
  BuzzerSwOnFltShortHigh_enum : Constant  Value=0
  BuzzerSwOnFltShortLow_enum : Constant  Value=0
  EEPROMFault_enum : Constant  Value=0
  LampBlueOnFltOpenCircuit_enum : Constant  Value=0
  LampBuleOnFltShortHigh_enum : Constant  Value=0
  LampBuleOnFltShortLow_enum : Constant  Value=0
  LampGreenOnFltOpenCircuit_enum : Constant  Value=0
  LampGreenOnFltShortHigh_enum : Constant  Value=0
  LampGreenOnFltShortLow_enum : Constant  Value=0
  LampRedOnFltOpenCircuit_enum : Constant  Value=0
  LampRedOnFltShortHigh_enum : Constant  Value=0
  LampRedOnFltShortLow_enum : Constant  Value=0
  LampYellowOnFltOpenCircuit_enum : Constant  Value=0
  LampYellowOnFltShortHigh_enum : Constant  Value=0
  LampYellowOnFltShortLow_enum : Constant  Value=0
  OBUBuzzerOnFltOpenCircuit_enum : Constant  Value=0
  OBUBuzzerOnFltShortHigh_enum : Constant  Value=0
  OBUBuzzerOnFltShortLow_enum : Constant  Value=0
  RAMFault_enum : Constant  Value=0
  ROMFault_enum : Constant  Value=0
  VREF1Fault_enum : Constant  Value=0
  VREF2Fault_enum : Constant  Value=0
  VHAL_AppTime_ms : Outport
  VHAL_ADCFault_enum : Outport  Port=2
  VHAL_EEPROMFault_enum : Outport  Port=3
  VHAL_RAMFault_enum : Outport  Port=4
  VHAL_ROMFault_enum : Outport  Port=5
  VHAL_VREF1Fault_enum : Outport  Port=6
  VHAL_VREF2Fault_enum : Outport  Port=7
  VHAL_BuzzerSwOnFltOpenCircuit_enum : Outport  Port=8
  VHAL_BuzzerSwOnFltShortHigh_enum : Outport  Port=9
  VHAL_BuzzerSwOnFltShortLow_enum : Outport  Port=10
  VHAL_OBUBuzzerOnFltOpenCircuit_enum : Outport  Port=11
  VHAL_OBUBuzzerOnFltShortHigh_enum : Outport  Port=12
  VHAL_OBUBuzzerOnFltShortLow_enum : Outport  Port=13
  VHAL_LampRedOnFltOpenCircuit_enum : Outport  Port=14
  VHAL_LampRedOnFltShortHigh_enum : Outport  Port=15
  VHAL_LampRedOnFltShortLow_enum : Outport  Port=16
  VHAL_LampBlueOnFltOpenCircuit_enum : Outport  Port=17
  VHAL_LampBuleOnFltShortHigh_enum : Outport  Port=18
  VHAL_LampBuleOnFltShortLow_enum : Outport  Port=19
  VHAL_LampGreenOnFltOpenCircuit_enum : Outport  Port=20
  VHAL_LampGreenOnFltShortHigh_enum : Outport  Port=21
  VHAL_LampGreenOnFltShortLow_enum : Outport  Port=22
  VHAL_LampYellowOnFltOpenCircuit_enum : Outport  Port=23
  VHAL_LampYellowOnFltShortHigh_enum : Outport  Port=24
  VHAL_LampYellowOnFltShortLow_enum : Outport  Port=25
  wires:
  VREF2Fault_enum/1 -> VHAL_VREF2Fault_enum/1
  VREF1Fault_enum/1 -> VHAL_VREF1Fault_enum/1
  ROMFault_enum/1 -> VHAL_ROMFault_enum/1
  RAMFault_enum/1 -> VHAL_RAMFault_enum/1
  EEPROMFault_enum/1 -> VHAL_EEPROMFault_enum/1
  AppTime_ms/1 -> VHAL_AppTime_ms/1
  ADCFault_enum/1 -> VHAL_ADCFault_enum/1
  BuzzerSwOnFltOpenCircuit_enum/1 -> VHAL_BuzzerSwOnFltOpenCircuit_enum/1
  BuzzerSwOnFltShortHigh_enum/1 -> VHAL_BuzzerSwOnFltShortHigh_enum/1
  BuzzerSwOnFltShortLow_enum/1 -> VHAL_BuzzerSwOnFltShortLow_enum/1
  OBUBuzzerOnFltOpenCircuit_enum/1 -> VHAL_OBUBuzzerOnFltOpenCircuit_enum/1
  OBUBuzzerOnFltShortHigh_enum/1 -> VHAL_OBUBuzzerOnFltShortHigh_enum/1
  OBUBuzzerOnFltShortLow_enum/1 -> VHAL_OBUBuzzerOnFltShortLow_enum/1
  LampRedOnFltOpenCircuit_enum/1 -> VHAL_LampRedOnFltOpenCircuit_enum/1
  LampRedOnFltShortHigh_enum/1 -> VHAL_LampRedOnFltShortHigh_enum/1
  LampRedOnFltShortLow_enum/1 -> VHAL_LampRedOnFltShortLow_enum/1
  LampBlueOnFltOpenCircuit_enum/1 -> VHAL_LampBlueOnFltOpenCircuit_enum/1
  LampBuleOnFltShortHigh_enum/1 -> VHAL_LampBuleOnFltShortHigh_enum/1
  LampBuleOnFltShortLow_enum/1 -> VHAL_LampBuleOnFltShortLow_enum/1
  LampGreenOnFltOpenCircuit_enum/1 -> VHAL_LampGreenOnFltOpenCircuit_enum/1
  LampGreenOnFltShortHigh_enum/1 -> VHAL_LampGreenOnFltShortHigh_enum/1
  LampGreenOnFltShortLow_enum/1 -> VHAL_LampGreenOnFltShortLow_enum/1
  LampYellowOnFltOpenCircuit_enum/1 -> VHAL_LampYellowOnFltOpenCircuit_enum/1
  LampYellowOnFltShortHigh_enum/1 -> VHAL_LampYellowOnFltShortHigh_enum/1
  LampYellowOnFltShortLow_enum/1 -> VHAL_LampYellowOnFltShortLow_enum/1

== system hcu_main_ADASwEPS/dHAL_IN/dHAL_IN_METER ==
  CAN1_Rx : Inport
  BO__1104_Meter1__8_Meter : Subsystem
  BO__1306_Meter3__8_Meter : Subsystem
  KFUN_AStpTimeMin_s1 : Constant  Value=INVALID_METER_VEHSPD
  KFUN_AStpTimeMin_s5 : Constant  Value=INVALID_ODO_METER
  Meter_Ind_VehSpeed_cvt : Subsystem  mask(ConvertOut){gain=0.125, offset=0}
      mask help:
      | Conversion Formula
      |
      | The conversion formula is
      |
      | raw_value = (physical_value - Offset) / Factor
      |
      | where physical_value is the value of the signal after it is saturated using the specified Min and Max values. raw_value is the packed signal value.
  ODOMETER_cvt : Subsystem  mask(ConvertOut){gain=1, offset=0}
      mask help:
      | Conversion Formula
      |
      | The conversion formula is
      |
      | raw_value = (physical_value - Offset) / Factor
      |
      | where physical_value is the value of the signal after it is saturated using the specified Min and Max values. raw_value is the packed signal value.
  Relational Operator1 : RelationalOperator  OutDataTypeStr=boolean
  Relational Operator4 : RelationalOperator  OutDataTypeStr=boolean
  VHAL_OdoMeter_km : Outport
  VHAL_OdoMeterInvalid_flg : Outport  Port=2
  VHAL_LowBrakeFluid_flg : Outport  Port=3
  VHAL_ParkBrakeOn_flg : Outport  Port=4
  VHAL_SeatBeltNOTFasten_flg : Outport  Port=5
  VHAL_MeterVehSpd_kph : Outport  Port=6
  VHAL_MeterVehSpdInvalid_flg : Outport  Port=7
  wires:
  BO__1104_Meter1__8_Meter/4(SeatBelt) -> VHAL_SeatBeltNOTFasten_flg/1
  BO__1104_Meter1__8_Meter/3(ParkBrake) -> VHAL_ParkBrakeOn_flg/1
  BO__1104_Meter1__8_Meter/1(LowBrakeFluid_Sta) -> VHAL_LowBrakeFluid_flg/1
  CAN1_Rx/1 -> [CAN1_Rx]
  [CAN1_Rx] -> BO__1104_Meter1__8_Meter/1(CAN1_Rx)
  [CAN1_Rx] -> BO__1306_Meter3__8_Meter/1(CAN1_Rx)
  BO__1104_Meter1__8_Meter/2(ODOMETER) -> ODOMETER_cvt/1(value), VHAL_OdoMeter_km/1
  KFUN_AStpTimeMin_s5/1 -> Relational Operator4/2
  ODOMETER_cvt/1(raw32) -> Relational Operator4/1
  Relational Operator4/1 -> VHAL_OdoMeterInvalid_flg/1
  BO__1306_Meter3__8_Meter/1(Meter_Ind_VehSpeed) -> Meter_Ind_VehSpeed_cvt/1(value), VHAL_MeterVehSpd_kph/1
  KFUN_AStpTimeMin_s1/1 -> Relational Operator1/2
  Meter_Ind_VehSpeed_cvt/1(raw32) -> Relational Operator1/1
  Relational Operator1/1 -> VHAL_MeterVehSpdInvalid_flg/1

== system hcu_main_ADASwEPS/dHAL_IN/dHAL_IN_TCM ==
  CAN1_Rx : Inport
  BO__832_TCM1__8_TCM : Subsystem
  BO__842_TCM2__8_TCM : Subsystem
  KFUN_AStpTimeMin_s3 : Constant  Value=INVALID_SHIFTER_POSN
  Relational Operator3 : RelationalOperator  Operator===  OutDataTypeStr=boolean
  VHAL_ShifterPosn_enum : Outport
  VHAL_ShifterPosnInvalid_flg : Outport  Port=2
  VHAL_NowGearPosn_enum : Outport  Port=3
  VHAL_NowGearPosnInvalid_flg : Outport  Port=4
  VHAL_TMTurbineSpd_rpm : Outport  Port=5
  VHAL_TMTurbineSpdInvalid_flg : Outport  Port=6
  VHAL_TqConvClutchSt_enum : Outport  Port=7
  VHAL_TCMMILReq_flg : Outport  Port=8
  VHAL_TCMWinterMode_flg : Outport  Port=9
  VHAL_TCMPowerMode_flg : Outport  Port=10
  VHAL_TCMFaultStatus_enum : Outport  Port=11
  VHAL_DriverMode_enum : Outport  Port=12
  wires:
  BO__842_TCM2__8_TCM/1(DR_MODE_IND) -> VHAL_DriverMode_enum/1
  BO__832_TCM1__8_TCM/1(CAN_ETCU_STATE) -> VHAL_TCMFaultStatus_enum/1
  BO__832_TCM1__8_TCM/6(LV_CAN_N_TM_ERR) -> VHAL_TMTurbineSpdInvalid_flg/1
  BO__832_TCM1__8_TCM/5(CAN_N_TM) -> VHAL_TMTurbineSpd_rpm/1
  BO__832_TCM1__8_TCM/4(CAN_GEAR_STA_NOW_V) -> VHAL_NowGearPosnInvalid_flg/1
  BO__832_TCM1__8_TCM/3(CAN_GEAR_STATE_NOW) -> VHAL_NowGearPosn_enum/1
  Relational Operator3/1 -> VHAL_ShifterPosnInvalid_flg/1
  KFUN_AStpTimeMin_s3/1 -> Relational Operator3/2
  BO__832_TCM1__8_TCM/2(CAN_GEAR_SEL_ETCU) -> Relational Operator3/1, VHAL_ShifterPosn_enum/1
  CAN1_Rx/1 -> [CAN1_Rx]
  [CAN1_Rx] -> BO__832_TCM1__8_TCM/1(CAN1_Rx)
  [CAN1_Rx] -> BO__842_TCM2__8_TCM/1(CAN1_Rx)
  BO__832_TCM1__8_TCM/7(CAN_SWI_CC_ETCU) -> VHAL_TqConvClutchSt_enum/1
  BO__832_TCM1__8_TCM/8(CAN_ETCU_OBD) -> VHAL_TCMMILReq_flg/1
  BO__832_TCM1__8_TCM/9(CAN_WTR) -> VHAL_TCMWinterMode_flg/1
  BO__832_TCM1__8_TCM/10(CAN_PWR) -> VHAL_TCMPowerMode_flg/1

== system hcu_main_ADASwEPS/EPSS/EPSS/AngleMode ==
  VEPSS_EPSTqOnShaftFlt_Nm : Inport
  VISP_StrAng_deg : Inport  Port=2
  VDINR_VehSpd_kph : Inport  Port=3
  VISP_StrAngReq_deg : Inport  Port=4
  VISP_StrAngReqAppl_flg : Inport  Port=5
  VISP_EPSModeReq_enum : Inport  Port=6
  VISP_ADASLFCStatus_enum : Inport  Port=7
  VISP_LFCTransGain_rat : Inport  Port=8
  VISP_LFCTransGainAppl_flg : Inport  Port=9
  Angle2Torque : Subsystem
  Constant : Constant  Value=-0.05
  Constant12 : Constant  Value=0.05
  Constant13 : Constant  Value=ENUM_EPSLFCSTATUS_TRANSITION
  Constant4 : Constant  Value=ENUM_EPSLFCSTATUS_ACTIVE
  IsInRange : hcu_lib/IsInRange  SystemSampleTime=-1
  LFC_Flow_Chart : Stateflow chart  TreatAsAtomicUnit=on
  Logical Operator1 : Logic  Operator=OR  AllPortsSameDT=off  OutDataTypeStr=boolean
  Relational Operator7 : RelationalOperator  Operator===  OutDataTypeStr=boolean
  Relational Operator8 : RelationalOperator  Operator===  OutDataTypeStr=boolean
  Switch4 : Switch  Criteria=u2 ~= 0
  VEPSS_StrWhlTqReqAng_Nm : Outport
  VEPSS_AngleModeActive_flg : Outport  Port=2
  VEPSS_EPSLFCStatus_enum : Outport  Port=3
  VEPSS_EPSLFCAbReason_enum : Outport  Port=4
  wires:
  [VEPSS_AngleModeActive_flg] -> VEPSS_AngleModeActive_flg/1  "VEPSS_AngleModeActive_flg"
  [VEPSS_EPSTqOnShaftFlt_Nm] -> Switch4/3
  [VEPSS_AngleModeActive_flg] -> Switch4/2
  [VEPSS_StrWhlTqReqAngRaw_Nm] -> Switch4/1
  VEPSS_EPSTqOnShaftFlt_Nm/1 -> Angle2Torque/2(VEPSS_EPSTqOnShaftFlt_Nm), [VEPSS_EPSTqOnShaftFlt_Nm]
  Switch4/1 -> VEPSS_StrWhlTqReqAng_Nm/1  "VEPSS_StrWhlTqReqAng_Nm"
  VISP_StrAngReq_deg/1 -> [VISP_StrAngReq_deg], Angle2Torque/4(VISP_StrAngReq_deg)
  VISP_StrAng_deg/1 -> Angle2Torque/1(VISP_StrAng_deg)
  VDINR_VehSpd_kph/1 -> Angle2Torque/3(VDINR_VehSpd_kph)
  [VEPSS_AngleModeActive_flg] -> Angle2Torque/8(VEPSS_AngleModeActive_flg)
  Angle2Torque/1(VEPSS_StrWhlTqReqAngRaw_Nm) -> [VEPSS_StrWhlTqReqAngRaw_Nm]
  [VEPSS_EPSLFCStatus_enum] -> Angle2Torque/7(VEPSS_EPSLFCStatus_enum)
  VISP_LFCTransGain_rat/1 -> Angle2Torque/5(VISP_LFCTransGain_rat)
  VISP_LFCTransGainAppl_flg/1 -> Angle2Torque/6(VISP_LFCTransGainAppl_flg)
  [VISP_StrAngReq_deg] -> IsInRange/1
  IsInRange/1 -> [VEPSS_StrAngReqZERO_flg]
  Constant/1 -> IsInRange/3
  Constant12/1 -> IsInRange/2
  LFC_Flow_Chart/1(VEPSS_EPSLFCStatus_enum) -> [VEPSS_EPSLFCStatus_enum], VEPSS_EPSLFCStatus_enum/1, Relational Operator8/1, Relational Operator7/1
  Constant4/1 -> Relational Operator7/2
  Constant13/1 -> Relational Operator8/2
  LFC_Flow_Chart/2(VEPSS_EPSLFCAbReason_enum) -> VEPSS_EPSLFCAbReason_enum/1
  Relational Operator8/1 -> Logical Operator1/2
  Relational Operator7/1 -> Logical Operator1/1
  Logical Operator1/1 -> [VEPSS_AngleModeActive_flg]
  VISP_ADASLFCStatus_enum/1 -> LFC_Flow_Chart/1(VISP_ADASLFCStatus_enum)
  VISP_EPSModeReq_enum/1 -> LFC_Flow_Chart/2(VISP_EPSModeReq_enum)
  VISP_StrAngReqAppl_flg/1 -> LFC_Flow_Chart/3(VISP_StrAngReqAppl_flg)
  [VEPSS_StrAngReqZERO_flg] -> LFC_Flow_Chart/4(VEPSS_StrAngReqZERO_flg)

== system hcu_main_ADASwEPS/EPSS/EPSS/EPSMotorPWMRequest ==
  VEPSS_StrWhlTqReqAst_Nm : Inport
  VEPSS_StrWhlTqReqTq_Nm : Inport  Port=2
  VEPSS_StrWhlTqReqAng_Nm : Inport  Port=3
  VEPSS_EPSLFCStatus_enum : Inport  Port=4
  VEPSS_TorqueModeActive_flg : Inport  Port=5
  VEPSS_AngleModeActive_flg : Inport  Port=6
  VISP_VehSpd_kph : Inport  Port=7
  VISP_LFCTransGain_rat : Inport  Port=8
  VISP_LFCTransGainAppl_flg : Inport  Port=9
  VISP_EPSModeReq_enum : Inport  Port=10
  VISP_EPSTqOnShaftValid_flg : Inport  Port=11
  EPSControl_Off : Constant  Value=0
  MotorPWMRequestCalculation : Subsystem
  MotorTorqueRequestCalculation : Subsystem
  Switch2 : Switch  Criteria=u2 ~= 0
  VEPSS_EPSMotPWMReq_pct : Outport
  wires:
  EPSControl_Off/1 -> Switch2/3
  VEPSS_EPSLFCStatus_enum/1 -> MotorTorqueRequestCalculation/9(VEPSS_EPSLFCStatus_enum)
  Switch2/1 -> VEPSS_EPSMotPWMReq_pct/1  "VEPSS_EPSMotPWMReq_pct"
  MotorTorqueRequestCalculation/1(VEPSS_EPSMotTqReq_Nm) -> MotorPWMRequestCalculation/1(VEPSS_EPSMotTqReqRaw_Nm)
  VISP_EPSTqOnShaftValid_flg/1 -> Switch2/2
  VEPSS_StrWhlTqReqAst_Nm/1 -> MotorTorqueRequestCalculation/1(VEPSS_StrWhlTqReqAst_Nm)
  VEPSS_StrWhlTqReqTq_Nm/1 -> MotorTorqueRequestCalculation/2(VEPSS_StrWhlTqReqTq_Nm)
  VEPSS_StrWhlTqReqAng_Nm/1 -> MotorTorqueRequestCalculation/3(VEPSS_StrWhlTqReqAng_Nm)
  VEPSS_TorqueModeActive_flg/1 -> MotorTorqueRequestCalculation/4(VEPSS_TorqueModeActive_flg)
  VEPSS_AngleModeActive_flg/1 -> MotorTorqueRequestCalculation/5(VEPSS_AngleModeActive_flg)
  VISP_VehSpd_kph/1 -> MotorTorqueRequestCalculation/6(VISP_VehSpd_kph)
  VISP_LFCTransGain_rat/1 -> MotorTorqueRequestCalculation/7(VISP_LFCTransGain_rat)
  VISP_LFCTransGainAppl_flg/1 -> MotorTorqueRequestCalculation/8(VISP_LFCTransGainAppl_flg)
  MotorPWMRequestCalculation/1(VEPSS_EPSMotPWMReqRaw_pct) -> Switch2/1
  VISP_EPSModeReq_enum/1 -> MotorTorqueRequestCalculation/10(VISP_EPSModeReq_enum)

== system hcu_main_ADASwEPS/EPSS/EPSS/EPSTest ==
  PassThrough : Inport
  Amplitude_pct : Constant  Value=5
  Compare To Constant : simulink/Logic and Bit Operations/Compare To Constant  relop===  const=3.0  OutDataTypeStr=boolean
  Constant : Constant  Value=2*pi  OutDataTypeStr=single
  Frequency_Hz : Constant
  Multiport Switch1 : MultiPortSwitch  Inputs=4
  PWMSetPt : Constant
  Product : Product  Inputs=3  RndMeth=Zero
  Product1 : Product  RndMeth=Zero
  SignalPlayer : Subsystem
  TestMode_Sw : Constant
  Timer : Subsystem
  Trigonometric Funcon : Trigonometry
  PWMOut : Outport
  wires:
  Multiport Switch1/1 -> PWMOut/1  "PWMOut"
  PassThrough/1 -> Multiport Switch1/2
  PWMSetPt/1 -> Multiport Switch1/3
  Product1/1 -> Multiport Switch1/4
  Frequency_Hz/1 -> Product/2
  Product/1 -> Trigonometric Funcon/1
  Amplitude_pct/1 -> Product1/2
  Trigonometric Funcon/1 -> Product1/1
  Constant/1 -> Product/3
  Timer/1(SineTime_s) -> Product/1
  TestMode_Sw/1 -> SignalPlayer/1(In1), Compare To Constant/1, Multiport Switch1/1
  Compare To Constant/1 -> Timer/Enable
  SignalPlayer/1(Out1) -> Multiport Switch1/5

== system hcu_main_ADASwEPS/EPSS/EPSS/InternalMode ==
  VEPSS_EPSTqOnShaftFlt_Nm : Inport
  VISP_StrTqReq_Nm : Inport  Port=2
  VISP_StrTqReqAppl_flg : Inport  Port=3
  VISP_EPSModeReq_enum : Inport  Port=4
  VISP_ADASLKAStatus_enum : Inport  Port=5
  Constant : Constant  Value=-0.05
  Constant1 : Constant  Value=0.05
  Constant5 : Constant  Value=ENUM_EPSLKASTATUS_ACTIVE
  IsInRange : hcu_lib/IsInRange  SystemSampleTime=-1
  LKA_Flow_Chart : Stateflow chart  TreatAsAtomicUnit=on
  Relational Operator2 : RelationalOperator  Operator===  OutDataTypeStr=boolean
  Sum : Sum
  Switch4 : Switch  Criteria=u2 ~= 0
  VEPSS_StrWhlTqReqAst_Nm : Outport
  VEPSS_EPSLKAStatus_enum : Outport  Port=2
  VEPSS_EPSLKAAbReason_enum : Outport  Port=3
  wires:
  VEPSS_EPSTqOnShaftFlt_Nm/1 -> Sum/2, Switch4/3
  Constant5/1 -> Relational Operator2/2
  [VEPSS_EPSLKAStatus_enum] -> Relational Operator2/1
  VISP_StrTqReq_Nm/1 -> IsInRange/1, Sum/1
  Switch4/1 -> VEPSS_StrWhlTqReqAst_Nm/1  "VEPSS_StrWhlTqReqAst_Nm"
  LKA_Flow_Chart/1(VEPSS_EPSLKAStatus_enum) -> [VEPSS_EPSLKAStatus_enum], VEPSS_EPSLKAStatus_enum/1
  Relational Operator2/1 -> Switch4/2
  Sum/1 -> Switch4/1
  LKA_Flow_Chart/2(VEPSS_EPSLKAAbReason_enum) -> VEPSS_EPSLKAAbReason_enum/1
  VISP_ADASLKAStatus_enum/1 -> LKA_Flow_Chart/1(VISP_ADASLKAStatus_enum)
  VISP_EPSModeReq_enum/1 -> LKA_Flow_Chart/2(VISP_EPSModeReq_enum)
  VISP_StrTqReqAppl_flg/1 -> LKA_Flow_Chart/4(VISP_StrTqReqAppl_flg)
  IsInRange/1 -> [VEPSS_StrTqReqZERO_flg]
  [VEPSS_StrTqReqZERO_flg] -> LKA_Flow_Chart/3(VEPSS_StrTqReqZERO_flg)
  Constant/1 -> IsInRange/3
  Constant1/1 -> IsInRange/2

== system hcu_main_ADASwEPS/EPSS/EPSS/InverseAssistTable ==
  1/KSTR_PWM2TqGain_rat : Gain
  MSTR_EPSMotPWMRescalingInv_pct : Lookup  InputValues=[-250 -3 0 3 250]  Table=[-100 -3 0 3 100]  LookUpMeth=Interpolation-Use End Values
      settings: AttributesFormatString="Input=\"%<InputValues>\"\\nOutput=\"%<Table>\""
  MSTR_TqAssistPWM_pct : Lookup  InputValues="[-100\t-95\t-90\t-85\t-80\t-75\t-70\t-65\t-60\t-55\t-50\t-45\t-40\t-35\t-30\t-25\t-20\t-15\t-10\t-5\t0\t5\t10\t15\t20\t25\t30\t35\t40\t45\t50\t55\t60\t65\t70\t75\t80\t85\t90\t95\t100]"  Table=[-10:0.5:10]  LookUpMeth=Interpolation-Use End Values
      settings: AttributesFormatString="Input=\"%<InputValues>\"\\nOutput=\"%<Table>\""
  MSTR_VehSpdPWMMult_rat : Lookup  InputValues=[-100 -80 -60 -40 -20 -10 0 10 20 40 60 80 100]  Table=[1 1 1 1 1 1 1 1 1 1 1 1 1]  LookUpMeth=Interpolation-Use End Values
      settings: AttributesFormatString="Input=\"%<InputValues>\"\\nOutput=\"%<Table>\""
  Product : Product  Inputs=*/
  Terminator : Terminator
  Terminator1 : Terminator
  VDINR_VehSpd_kph : Constant  Value=0
  VSTR_EPSMotTqReq_Nm : Constant  Value=0
  wires:
  MSTR_EPSMotPWMRescalingInv_pct/1 -> Product/1
  VSTR_EPSMotTqReq_Nm/1 -> 1/KSTR_PWM2TqGain_rat/1
  1/KSTR_PWM2TqGain_rat/1 -> Terminator1/1, MSTR_EPSMotPWMRescalingInv_pct/1  "PWMInput"
  VDINR_VehSpd_kph/1 -> MSTR_VehSpdPWMMult_rat/1
  MSTR_VehSpdPWMMult_rat/1 -> Product/2
  Product/1 -> MSTR_TqAssistPWM_pct/1
  MSTR_TqAssistPWM_pct/1 -> Terminator/1  "VSTR_StrWheelTqReq_Nm"
